simulink subsystem "rss_StrtUpPrcdChkNeed"  (R2023a)
settings: Solver=VariableStepAuto  StartTime=0.0  StopTime=10.0  RelTol=1e-3
undefined symbols (not defined in the file): Cdbl_nElecAgSpdMaxVal, ENM_MOTO_STATUS, Gs16_nMinStrtUpElecSpd_C, Gs16_nStrtUpProcTolcElecSpd_C
libraries: lib_conversion x2, simulink x1, lib_moving_average_filter x1
settings Model: Creator=xiaoqiang.yuan  LastModifiedBy=xiaoqiang.yuan

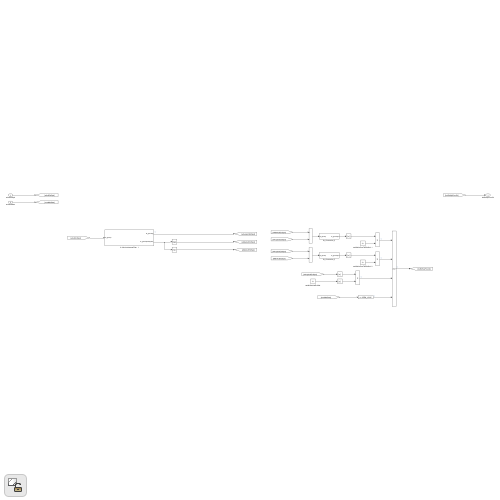
[thumbnail: Simulink's stored preview of the top-level diagram]
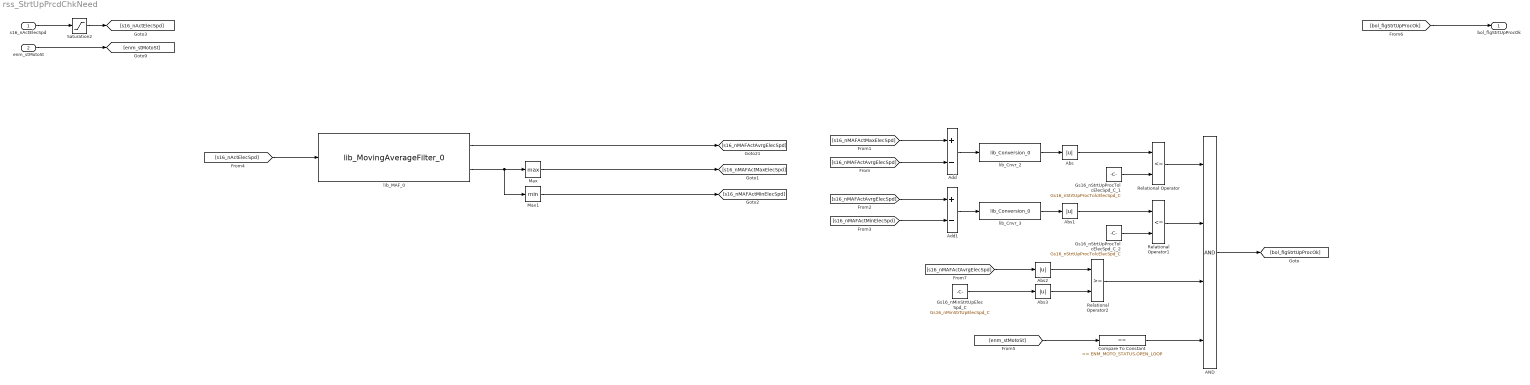
== system rss_StrtUpPrcdChkNeed ==
  s16_nActElecSpd : Inport  OutDataTypeStr=dt_Standardize_s16p15b0  PortDimensions=1
  enm_stMotoSt : Inport  Port=2  OutDataTypeStr=Enum: ENM_MOTO_STATUS
  AND : Logic  Inputs=4  AllPortsSameDT=off  OutDataTypeStr=boolean
  Abs{,1..3} (4 alike) : Abs  SaturateOnIntegerOverflow=off
  Add : Sum  Inputs=+-  OutDataTypeStr=Inherit: Inherit via back propagation
  Add1 : Sum  Inputs=+-  OutDataTypeStr=Inherit: Inherit via back propagation
  Compare To Constant : simulink/Logic and Bit Operations/Compare To Constant  relop===  const=ENM_MOTO_STATUS.OPEN_LOOP  OutDataTypeStr=boolean
  Gs16_nMinStrtUpElecSpd_C : Constant  Value=Gs16_nMinStrtUpElecSpd_C
  Gs16_nStrtUpProcTolcElecSpd_C_1 : Constant  Value=Gs16_nStrtUpProcTolcElecSpd_C
  Gs16_nStrtUpProcTolcElecSpd_C_2 : Constant  Value=Gs16_nStrtUpProcTolcElecSpd_C
  Max : MinMax  Function=max  OutDataTypeStr=Inherit: Same as first input
  Max1 : MinMax  OutDataTypeStr=Inherit: Same as first input
  Relational Operator : RelationalOperator  Operator=<=  OutDataTypeStr=boolean  RndMeth=Simplest  InputSameDT=off
  Relational Operator1 : RelationalOperator  Operator=<=  OutDataTypeStr=boolean  RndMeth=Simplest  InputSameDT=off
  Relational Operator2 : RelationalOperator  OutDataTypeStr=boolean  RndMeth=Simplest  InputSameDT=off
  Saturation2 : Saturate  UpperLimit=Cdbl_nElecAgSpdMaxVal  LowerLimit=-Cdbl_nElecAgSpdMaxVal
  lib_Cnvr_2 : lib_conversion/lib_Conversion_0  lb_parDataType=dt_Standardize_s16p15b0  lb_parOutpMaxVal=[]  lb_parOutpMinVal=[]  lb_parSatFlag=off
  lib_Cnvr_3 : lib_conversion/lib_Conversion_0  lb_parDataType=dt_Standardize_s16p15b0  lb_parOutpMaxVal=[]  lb_parOutpMinVal=[]  lb_parSatFlag=off
  lib_MAF_0 : lib_moving_average_filter/lib_MovingAverageFilter_0  lb_parSampNum=20  lb_parInpSmtnDataType=fixdt(1,32,2^-14,0)
  bol_flgStrtUpProcOk : Outport  OutDataTypeStr=boolean
  wires:
  Relational Operator2/1 -> AND/3
  [bol_flgStrtUpProcOk] -> bol_flgStrtUpProcOk/1
  [enm_stMotoSt] -> Compare To Constant/1
  lib_MAF_0/1 -> [s16_nMAFActAvrgElecSpd]
  AND/1 -> [bol_flgStrtUpProcOk]
  [s16_nActElecSpd] -> lib_MAF_0/1
  Abs2/1 -> Relational Operator2/1
  Max/1 -> [s16_nMAFActMaxElecSpd]
  lib_MAF_0/2 -> Max/1, Max1/1
  [s16_nMAFActAvrgElecSpd] -> Abs2/1
  s16_nActElecSpd/1 -> Saturation2/1
  enm_stMotoSt/1 -> [enm_stMotoSt]
  Abs1/1 -> Relational Operator1/1
  Gs16_nStrtUpProcTolcElecSpd_C_2/1 -> Relational Operator1/2
  Relational Operator/1 -> AND/1
  lib_Cnvr_3/1 -> Abs1/1
  Gs16_nMinStrtUpElecSpd_C/1 -> Abs3/1
  Add/1 -> lib_Cnvr_2/1
  Add1/1 -> lib_Cnvr_3/1
  Abs3/1 -> Relational Operator2/2
  Abs/1 -> Relational Operator/1
  Compare To Constant/1 -> AND/4
  [s16_nMAFActMinElecSpd] -> Add1/2
  [s16_nMAFActAvrgElecSpd] -> Add1/1
  lib_Cnvr_2/1 -> Abs/1
  [s16_nMAFActAvrgElecSpd] -> Add/2
  [s16_nMAFActMaxElecSpd] -> Add/1
  Max1/1 -> [s16_nMAFActMinElecSpd]
  Relational Operator1/1 -> AND/2
  Gs16_nStrtUpProcTolcElecSpd_C_1/1 -> Relational Operator/2
  Saturation2/1 -> [s16_nActElecSpd]
